simulink model "Exercise4Pt2"  (R2019b)
settings: Solver=VariableStepAuto  StartTime=0.0  StopTime=3000  RelTol=1e-3
values from neighbouring files (symbols this model uses):
  a_in = 0    [NewtonsSecondLaw.m]
  a_out = 0    [NewtonsSecondLaw.m]
  c = 16    [NewtonsSecondLaw.m]
  K_out = 0.1587/60    (= 0.002645)    [NewtonsSecondLaw.m]
  Q_in = (10*0.134)/60    (= 0.0223333333333)    [NewtonsSecondLaw.m]
settings Model: Creator=dzecc  LastModifiedBy=dzecc

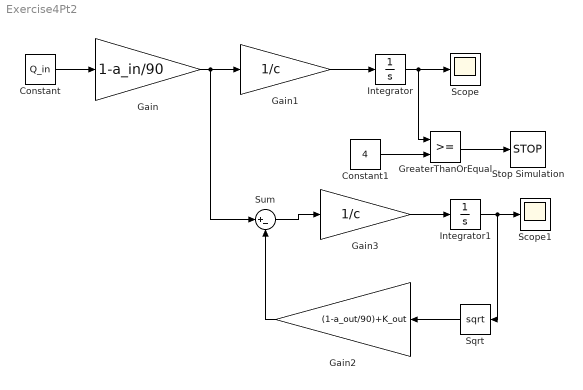
== system Exercise4Pt2 ==
  Constant : Constant  Value=Q_in  VectorParams1D=off
  Constant1 : Constant  Value=4
  Gain : Gain  Gain=1-a_in/90
  Gain1 : Gain  Gain=1/c
  Gain2 : Gain  Gain=(1-a_out/90)+K_out
  Gain3 : Gain  Gain=1/c
  GreaterThanOrEqual : RelationalOperator  OutDataTypeStr=boolean  RndMeth=Simplest
  Integrator : Integrator
  Integrator1 : Integrator
  Scope : Scope
  Scope1 : Scope
  Sqrt : Sqrt  SaturateOnIntegerOverflow=on
  Stop Simulation : Stop
  Sum : Sum  Inputs=|+-
  wires:
  Constant/1 -> Gain/1
  Gain/1 -> Sum/1, Gain1/1
  Gain1/1 -> Integrator/1
  Integrator/1 -> GreaterThanOrEqual/1, Scope/1
  GreaterThanOrEqual/1 -> Stop Simulation/1
  Constant1/1 -> GreaterThanOrEqual/2
  Sum/1 -> Gain3/1
  Gain3/1 -> Integrator1/1
  Integrator1/1 -> Sqrt/1, Scope1/1
  Sqrt/1 -> Gain2/1
  Gain2/1 -> Sum/2
